simulink model "Simulink_TEP"  (R2024a)
settings: Solver=FixedStepAuto  StartTime=0.0  StopTime=5  FixedStep=1/3600  RelTol=1e-3
model workspace (MAT data in the model file):
  AD : Simulink.Parameter (value not decoded)
  AG : Simulink.Parameter (value not decoded)
  AH : Simulink.Parameter (value not decoded)
  AV : Simulink.Parameter (value not decoded)
  AVP : Simulink.Parameter (value not decoded)
  BCHL : Simulink.Parameter (value not decoded)
  BCHV : Simulink.Parameter (value not decoded)
  BD : Simulink.Parameter (value not decoded)
  BG : Simulink.Parameter (value not decoded)
  BH : Simulink.Parameter (value not decoded)
  BVP : Simulink.Parameter (value not decoded)
  CD : Simulink.Parameter (value not decoded)
  CG : Simulink.Parameter (value not decoded)
  CH : Simulink.Parameter (value not decoded)
  CVP : Simulink.Parameter (value not decoded)
  XMW : Simulink.Parameter (value not decoded)
symbols that are objects in the model workspace (value not decoded): AD, AG, AH, AV, AVP, BD, BG, BH, BVP, CD, CG, CH, CVP, XMW
undefined symbols (not defined in the file or in its folder): magnitude, SETPT, XMEAS, XMV
libraries: mylib x165, dspindex x17
(part 4 of 10)

== system Simulink_TEP/Subsystem/Braatz ==
  XMEAS : Inport
  " " : Subsystem  mask{Parameter1=XMV(1), Parameter2=XMEAS(2), SETPT1=3664.0, GAIN1=1.0, SI1=3, HIGH1=5811, Parameter1_copy=SETPT(1), Parameter2_copy=XMEAS(26), SETPT14=6.8820, GAIN14=8.3, TAUI14=3168.0/3600, SI14=360, HIGH14=100}
      mask prompts: Parameter1 "Manipulated Variable"; Parameter2 "Process Variable"; SETPT1 "Setpoint"; GAIN1 "Controller Gain"; SI1 "Sampling Interval"; HIGH1 "High Limit"; Parameter1_copy "Manipulated Variable"; Parameter2_copy "Process Variable"; SETPT14 "Setpoint"; GAIN14 "Controller Gain"; TAUI14 "Integral Time Constant"; SI14 "Sampling Interval"; HIGH14 "High Limit"
      mask DialogControl DescGroupVar Prompt: Control Variables
      mask DialogControl DescTextVar Prompt: Enter the control variables needed
      mask DialogControl ParameterGroupVar Prompt: Control 1
      mask DialogControl Container3 Prompt: Control 14
  " 1" : Subsystem  mask{Parameter1=XMV(2), Parameter2=XMEAS(3), SETPT2=4509.3, GAIN2=1.0, SI2=3, HIGH2=8354, Parameter1_copy=SETPT(2), Parameter2_copy=XMEAS(27), SETPT15=18.776, GAIN15=2.37, TAUI15=5069/3600, SI15=360, HIGH15=100}
      mask prompts: Parameter1 "Manipulated Variable"; Parameter2 "Process Variable"; SETPT2 "Setpoint"; GAIN2 "Controller Gain"; SI2 "Sampling Interval"; HIGH2 "High Limit"; Parameter1_copy "Manipulated Variable"; Parameter2_copy "Process Variable"; SETPT15 "Setpoint"; GAIN15 "Controller Gain"; TAUI15 "Integral Time Constant"; SI15 "Sampling Interval"; HIGH15 "High Limit"
      mask DialogControl DescGroupVar Prompt: Control Variables
      mask DialogControl DescTextVar Prompt: Enter the control variables needed
      mask DialogControl ParameterGroupVar Prompt: Control 2
      mask DialogControl Container3 Prompt: Control 15
  " 10" : Subsystem  mask{Parameter1=XMV(6), Parameter2=XMEAS(10), SETPT6=0.33712, GAIN6=1.22, SI6=3, HIGH6=1, Parameter1_copy=SETPT(6), Parameter2_copy=XMEAS(30), SETPT19=13.823, GAIN19=-83.2/5/3, TAUI19=6336/3600, SI19=360, HIGH19=26}
      mask prompts: Parameter1 "Manipulated Variable"; Parameter2 "Process Variable"; SETPT6 "Setpoint"; GAIN6 "Controller Gain"; SI6 "Sampling Interval"; HIGH6 "High Limit"; Parameter1_copy "Manipulated Variable"; Parameter2_copy "Process Variable"; SETPT19 "Setpoint"; GAIN19 "Controller Gain"; TAUI19 "Integral Time Constant"; SI19 "Sampling Interval"; HIGH19 "High Limit"
      mask DialogControl DescGroupVar Prompt: Control Variables
      mask DialogControl DescTextVar Prompt: Enter the control variables needed
      mask DialogControl ParameterGroupVar Prompt: Control 6
      mask DialogControl Container3 Prompt: Control 19
  " 2" : Subsystem  mask{Parameter1=XMV(3), Parameter2=XMEAS(1), SETPT3=0.25052, GAIN3=1.0, SI3=3, HIGH3=1.017, Parameter1_copy=SETPT(3), Parameter2_copy=XMEAS(23), SETPT13=32.188, GAIN13=18, TAUI13=3168.0/3600, SI13=360, HIGH13=100}
      mask prompts: Parameter1 "Manipulated Variable"; Parameter2 "Process Variable"; SETPT3 "Setpoint"; GAIN3 "Controller Gain"; SI3 "Sampling Interval"; HIGH3 "High Limit"; Parameter1_copy "Manipulated Variable"; Parameter2_copy "Process Variable"; SETPT13 "Setpoint"; GAIN13 "Controller Gain"; TAUI13 "Integral Time Constant"; SI13 "Sampling Interval"; HIGH13 "High Limit"
      mask DialogControl DescGroupVar Prompt: Control Variables
      mask DialogControl DescTextVar Prompt: Enter the control variables needed
      mask DialogControl ParameterGroupVar Prompt: Control 3
      mask DialogControl Container3 Prompt: Control 13
  " 3" : Subsystem  mask{Parameter1=XMV(4), Parameter2=XMEAS(4), SETPT4=9.3477, GAIN4=1.0, SI4=3, HIGH4=15.25, Parameter1_copy=SETPT(4), Parameter2_copy=XMEAS(8), SETPT17=75, GAIN17=11.1/10, TAUI17=3168.0/3600, SI17=3, HIGH17=50}
      mask prompts: Parameter1 "Manipulated Variable"; Parameter2 "Process Variable"; SETPT4 "Setpoint"; GAIN4 "Controller Gain"; SI4 "Sampling Interval"; HIGH4 "High Limit"; Parameter1_copy "Manipulated Variable"; Parameter2_copy "Process Variable"; SETPT17 "Setpoint"; GAIN17 "Controller Gain"; TAUI17 "Integral Time Constant"; SI17 "Sampling Interval"; HIGH17 "High Limit"
      mask DialogControl DescGroupVar Prompt: Control Variables
      mask DialogControl DescTextVar Prompt: Enter the control variables needed
      mask DialogControl ParameterGroupVar Prompt: Control 4
      mask DialogControl Container3 Prompt: Control 17
  " 4" : Subsystem  mask{Parameter1_copy=XMV(5), Parameter2_copy=XMEAS(5), SETPT5=26.902, GAIN5=-0.083, TAUI5=1/3600, SI5=3, HIGH5=53}
      mask prompts: Parameter1_copy "Manipulated Variable"; Parameter2_copy "Process Variable"; SETPT5 "Setpoint"; GAIN5 "Controller Gain"; TAUI5 "Integral Time Constant"; SI5 "Sampling Interval"; HIGH5 "High Limit"
      mask DialogControl DescGroupVar Prompt: Control Variables
      mask DialogControl DescTextVar Prompt: Enter the control variables needed
      mask DialogControl Container3 Prompt: Control 5
  " 5" : Subsystem  mask{Parameter1_copy=XMV(7), Parameter2_copy=XMEAS(12), SETPT7=50, GAIN7=-2.06, SI7=3, HIGH7=70}
      mask prompts: Parameter1_copy "Manipulated Variable"; Parameter2_copy "Process Variable"; SETPT7 "Setpoint"; GAIN7 "Controller Gain"; SI7 "Sampling Interval"; HIGH7 "High Limit"
      mask DialogControl DescGroupVar Prompt: Control Variables
      mask DialogControl DescTextVar Prompt: Enter the control variables needed
      mask DialogControl Container3 Prompt: Control 7
  " 6" : Subsystem  mask{Parameter1_copy=XMV(8), Parameter2_copy=XMEAS(15), SETPT8=50, GAIN8=-1.62, SI8=3, HIGH8=70}
      mask prompts: Parameter1_copy "Manipulated Variable"; Parameter2_copy "Process Variable"; SETPT8 "Setpoint"; GAIN8 "Controller Gain"; SI8 "Sampling Interval"; HIGH8 "High Limit"
      mask DialogControl DescGroupVar Prompt: Control Variables
      mask DialogControl DescTextVar Prompt: Enter the control variables needed
      mask DialogControl Container3 Prompt: Control 8
  " 7" : Subsystem  mask{Parameter1_copy=XMV(11), Parameter2_copy=XMEAS(17), SETPT11=22.949, GAIN11=1.09, TAUI11=2600/3600, SI11=3, HIGH11=46}
      mask prompts: Parameter1_copy "Manipulated Variable"; Parameter2_copy "Process Variable"; SETPT11 "Setpoint"; GAIN11 "Controller Gain"; TAUI11 "Integral Time Constant"; SI11 "Sampling Interval"; HIGH11 "High Limit"
      mask DialogControl DescGroupVar Prompt: Control Variables
      mask DialogControl DescTextVar Prompt: Enter the control variables needed
      mask DialogControl Container3 Prompt: Control 11
  " 8" : Subsystem  mask{Parameter1=XMV(10), Parameter2=XMEAS(21), SETPT10=94.599, GAIN10=-0.156*10, TAUI10=1452/3600, SI10=3, HIGH10=150, Parameter1_copy=SETPT(10), Parameter2_copy=XMEAS(9), SETPT18=120.4, GAIN18=2.83*10, TAUI18=982/3600, SI18=3, HIGH18=150}
      mask prompts: Parameter1 "Manipulated Variable"; Parameter2 "Process Variable"; SETPT10 "Setpoint"; GAIN10 "Controller Gain"; TAUI10 "Integral Time Constant"; SI10 "Sampling Interval"; HIGH10 "High Limit"; Parameter1_copy "Manipulated Variable"; Parameter2_copy "Process Variable"; SETPT18 "Setpoint"; GAIN18 "Controller Gain"; TAUI18 "Integral Time Constant"; SI18 "Sampling Interval"; HIGH18 "High Limit"
      mask DialogControl DescGroupVar Prompt: Control Variables
      mask DialogControl DescTextVar Prompt: Enter the control variables needed
      mask DialogControl ParameterGroupVar Prompt: Control 10
      mask DialogControl Container3 Prompt: Control 18
  " 9" : Subsystem  mask{Parameter1=XMV(9), Parameter2=XMEAS(19), SETPT9=230.31, GAIN9=0.41, SI9=3, HIGH9=460, Parameter1_copy=SETPT(9), Parameter2_copy=XMEAS(18), SETPT16=65.731, GAIN16=1.69/10, TAUI16=236/3600, SI16=3, HIGH16=130, Parameter1_copy_copy=SETPT(16), Parameter2_copy_copy=XMEAS(38), SETPT20=0.83570, GAIN20=-16.3/5, TAUI20=12408/3600, SI20=900, HIGH20=1.6}
      mask prompts: Parameter1 "Manipulated Variable"; Parameter2 "Process Variable"; SETPT9 "Setpoint"; GAIN9 "Controller Gain"; SI9 "Sampling Interval"; HIGH9 "High Limit"; Parameter1_copy "Manipulated Variable"; Parameter2_copy "Process Variable"; SETPT16 "Setpoint"; GAIN16 "Controller Gain"; TAUI16 "Integral Time Constant"; SI16 "Sampling Interval"; HIGH16 "High Limit"; Parameter1_copy_copy "Manipulated Variable"; Parameter2_copy_copy "Process Variable"; SETPT20 "Setpoint"; GAIN20 "Controller Gain"; TAUI20 "Integral Time Constant"; SI20 "Sampling Interval"; HIGH20 "High Limit"
      mask DialogControl DescGroupVar Prompt: Control Variables
      mask DialogControl DescTextVar Prompt: Enter the control variables needed
      mask DialogControl ParameterGroupVar Prompt: Control 9
      mask DialogControl Container3 Prompt: Control 16
      mask DialogControl Container3_copy Prompt: Control 20
  Bus Creator : BusCreator  Inputs=12
  Constant11 : Constant  Value=XMV12_0
  XMV : Outport  VectorParamsAs1DForOutWhenUnconnected=off
  wires:
  " "/1(XMV(1)) -> Bus Creator/1  "XMV(1)"
  " 1"/1(XMV(2)) -> Bus Creator/2  "XMV(2)"
  " 2"/1(XMV(3)) -> Bus Creator/3  "XMV(3)"
  " 3"/1(XMV(4)) -> Bus Creator/4  "XMV(4)"
  " 4"/1(XMV(5)) -> Bus Creator/5  "XMV(5)"
  " 10"/1(XMV(6)) -> Bus Creator/6  "XMV(6)"
  " 5"/1(XMV(7)) -> Bus Creator/7  "XMV(7)"
  " 6"/1(XMV(8)) -> Bus Creator/8  "XMV(8)"
  " 9"/1(XMV(9)) -> Bus Creator/9  "XMV(9)"
  " 8"/1(XMV(10)) -> Bus Creator/10  "XMV(10)"
  " 7"/1(XMV(11)) -> Bus Creator/11  "XMV(11)"
  Constant11/1 -> Bus Creator/12  "XMV(12)"
  Bus Creator/1 -> XMV/1
  XMEAS/1 -> " 5"/1(XMEAS), " 9"/1(XMEAS), " 8"/1(XMEAS), " 7"/1(XMEAS), " 6"/1(XMEAS), " 10"/1(XMEAS), " 4"/1(XMEAS), " 3"/1(XMEAS), " 2"/1(XMEAS), " 1"/1(XMEAS), " "/1(XMEAS)

== system Simulink_TEP/Subsystem/If Action Subsystem ==
  In1 : Inport
  Action Port : ActionPort  ActionPortLabel=if(u1 == 1)
  Out1 : Outport  VectorParamsAs1DForOutWhenUnconnected=off
  wires:
  In1/1 -> Out1/1

== system Simulink_TEP/Subsystem/If Action Subsystem1 ==
  In1 : Inport
  Action Port : ActionPort  ActionPortLabel=elseif(u2 == 1)
  Out1 : Outport  VectorParamsAs1DForOutWhenUnconnected=off
  wires:
  In1/1 -> Out1/1

== system Simulink_TEP/Subsystem/If Action Subsystem2 ==
  In1 : Inport
  Action Port : ActionPort  ActionPortLabel=elseif( u3 == 1)
  Out1 : Outport  VectorParamsAs1DForOutWhenUnconnected=off
  wires:
  In1/1 -> Out1/1

== system Simulink_TEP/Subsystem/Open loop ==
  Bus Creator : BusCreator  Inputs=12
  Constant : Constant  Value=XMV1_0
  Constant1 : Constant  Value=XMV2_0
  Constant10 : Constant  Value=XMV11_0
  Constant11 : Constant  Value=XMV12_0
  Constant2 : Constant  Value=XMV3_0
  Constant3 : Constant  Value=XMV4_0
  Constant4 : Constant  Value=XMV5_0
  Constant5 : Constant  Value=XMV6_0
  Constant6 : Constant  Value=XMV7_0
  Constant7 : Constant  Value=XMV8_0
  Constant8 : Constant  Value=XMV9_0
  Constant9 : Constant  Value=XMV10_0
  XMV : Outport  VectorParamsAs1DForOutWhenUnconnected=off
  wires:
  Constant5/1 -> Bus Creator/6  "XMV(6)"
  Constant1/1 -> Bus Creator/2  "XMV(2)"
  Constant4/1 -> Bus Creator/5  "XMV(5)"
  Constant3/1 -> Bus Creator/4  "XMV(4)"
  Constant2/1 -> Bus Creator/3  "XMV(3)"
  Constant11/1 -> Bus Creator/12  "XMV(12)"
  Constant10/1 -> Bus Creator/11  "XMV(11)"
  Constant/1 -> Bus Creator/1  "XMV(1)"
  Constant9/1 -> Bus Creator/10  "XMV(10)"
  Constant8/1 -> Bus Creator/9  "XMV(9)"
  Constant6/1 -> Bus Creator/7  "XMV(7)"
  Bus Creator/1 -> XMV/1
  Constant7/1 -> Bus Creator/8  "XMV(8)"

== system Simulink_TEP/Subsystem/Ricker ==
  Bus Creator : BusCreator  Inputs=12
  Constant : Constant  Value=XMV1_0
  Constant1 : Constant  Value=XMV2_0
  Constant10 : Constant  Value=XMV11_0
  Constant11 : Constant  Value=XMV12_0
  Constant2 : Constant  Value=XMV3_0
  Constant3 : Constant  Value=XMV4_0
  Constant4 : Constant  Value=XMV5_0
  Constant5 : Constant  Value=XMV6_0
  Constant6 : Constant  Value=XMV7_0
  Constant7 : Constant  Value=XMV8_0
  Constant8 : Constant  Value=XMV9_0
  Constant9 : Constant  Value=XMV10_0
  XMV : Outport  VectorParamsAs1DForOutWhenUnconnected=off
  wires:
  Constant5/1 -> Bus Creator/6  "XMV(6)"
  Constant1/1 -> Bus Creator/2  "XMV(2)"
  Constant4/1 -> Bus Creator/5  "XMV(5)"
  Constant3/1 -> Bus Creator/4  "XMV(4)"
  Constant2/1 -> Bus Creator/3  "XMV(3)"
  Constant11/1 -> Bus Creator/12  "XMV(12)"
  Constant10/1 -> Bus Creator/11  "XMV(11)"
  Constant/1 -> Bus Creator/1  "XMV(1)"
  Constant9/1 -> Bus Creator/10  "XMV(10)"
  Constant8/1 -> Bus Creator/9  "XMV(9)"
  Constant6/1 -> Bus Creator/7  "XMV(7)"
  Bus Creator/1 -> XMV/1
  Constant7/1 -> Bus Creator/8  "XMV(8)"

== system Simulink_TEP/Subsystem/Subsystem ==
  OPL : Inport
  B : Inport  Port=2
  R : Inport  Port=3
  Assertion : Assertion  AssertionFailFcn=|  StopWhenAssertionFail=off
      | set_param(bdroot,'SimulationCommand','stop'),
      | disp(sprintf('\nSimulation stoped.')), msgbox({'Simulation will not run';'More than one loop selected'}, 'Shutdown','error')
  Constant3 : Constant  Value=2
  Relational Operator : RelationalOperator  Operator=<  OutDataTypeStr=boolean  RndMeth=Simplest  InputSameDT=off
  Sum of Elements : Sum  Inputs=+++
  wires:
  Sum of Elements/1 -> Relational Operator/1
  R/1 -> Sum of Elements/3
  OPL/1 -> Sum of Elements/1
  Relational Operator/1 -> Assertion/1
  Constant3/1 -> Relational Operator/2
  B/1 -> Sum of Elements/2

== system Simulink_TEP/Subsystem1/Subsystem ==
  Stream 6 : Inport
  Bus Creator : BusCreator  Inputs=2
  Bus Selector : BusSelector  OutputSignals=signal1.Phase,signal1.TST(6) = TST(7),signal1.XST(I;6) = XST(I;7),PTV,signal1.FTM(6) = FTM(7)
  Exergy Molar Flow : mylib/Exergy Molar Flow  SystemSampleTime=-1  VariantActivationTime=update diagram  AllowFlexibleInterface=on  Latency=0  AutoFrameSizeCalculation=off
  B1 : Outport  VectorParamsAs1DForOutWhenUnconnected=off
  wires:
  Bus Selector/4 -> Exergy Molar Flow/4  "<PTV>"
  Exergy Molar Flow/2 -> Bus Creator/2  "Bph1"
  Bus Selector/5 -> Exergy Molar Flow/5  "<FTM(6) = FTM(7)>"
  Bus Selector/2 -> Exergy Molar Flow/2  "<TST(6) = TST(7)>"
  Stream 6/1 -> Bus Selector/1
  Bus Creator/1 -> B1/1  "B1"
  Bus Selector/3 -> Exergy Molar Flow/3  "<XST(I;6) = XST(I;7)>"
  Exergy Molar Flow/1 -> Bus Creator/1  "Bch1"
  Bus Selector/1 -> Exergy Molar Flow/1  "<Phase>"

== system Simulink_TEP/Subsystem1/Subsystem1 ==
  Stream 8 : Inport
  Bus Creator1 : BusCreator  Inputs=2
  Bus Selector : BusSelector  OutputSignals=signal1.Phase,signal1.TST(8),signal1.XST(I;8),PTR,signal1.FTM(8)
  Exergy Molar Flow : mylib/Exergy Molar Flow  SystemSampleTime=-1  VariantActivationTime=update diagram  AllowFlexibleInterface=on  Latency=0  AutoFrameSizeCalculation=off
  B2 : Outport  VectorParamsAs1DForOutWhenUnconnected=off
  wires:
  Bus Selector/4 -> Exergy Molar Flow/4  "<PTR>"
  Bus Selector/5 -> Exergy Molar Flow/5  "<FTM(8)>"
  Bus Selector/2 -> Exergy Molar Flow/2  "<TST(8)>"
  Stream 8/1 -> Bus Selector/1
  Bus Selector/3 -> Exergy Molar Flow/3  "<XST(I;8)>"
  Bus Selector/1 -> Exergy Molar Flow/1  "<Phase>"
  Exergy Molar Flow/2 -> Bus Creator1/2  "Bph2"
  Bus Creator1/1 -> B2/1  "B2"
  Exergy Molar Flow/1 -> Bus Creator1/1  "Bch2"

== system Simulink_TEP/Subsystem1/Subsystem2 ==
  Stream 9 : Inport
  Bus Creator2 : BusCreator  Inputs=2
  Bus Selector : BusSelector  OutputSignals=signal2.Phase,signal2.TST(9),signal2.XST(I;9),PTS,signal2.FTM(9)
  Exergy Molar Flow : mylib/Exergy Molar Flow  SystemSampleTime=-1  VariantActivationTime=update diagram  AllowFlexibleInterface=on  Latency=0  AutoFrameSizeCalculation=off
  B3 : Outport  VectorParamsAs1DForOutWhenUnconnected=off
  wires:
  Bus Selector/4 -> Exergy Molar Flow/4  "<PTS>"
  Bus Selector/5 -> Exergy Molar Flow/5  "<FTM(9)>"
  Bus Selector/2 -> Exergy Molar Flow/2  "<TST(9)>"
  Stream 9/1 -> Bus Selector/1
  Bus Selector/3 -> Exergy Molar Flow/3  "<XST(I;9)>"
  Bus Selector/1 -> Exergy Molar Flow/1  "<Phase>"
  Exergy Molar Flow/1 -> Bus Creator2/1  "Bch3"
  Exergy Molar Flow/2 -> Bus Creator2/2  "Bph3"
  Bus Creator2/1 -> B3/1  "B3"

== system Simulink_TEP/Subsystem1/Subsystem3 ==
  Stream 10 : Inport
  Bus Creator3 : BusCreator  Inputs=2
  Bus Selector : BusSelector  OutputSignals=signal1.Phase,signal1.TST(10),signal1.XST(I;10),PTS,signal1.FTM(10)
  Exergy Molar Flow : mylib/Exergy Molar Flow  SystemSampleTime=-1  VariantActivationTime=update diagram  AllowFlexibleInterface=on  Latency=0  AutoFrameSizeCalculation=off
  B4 : Outport  VectorParamsAs1DForOutWhenUnconnected=off
  wires:
  Bus Selector/4 -> Exergy Molar Flow/4  "<PTS>"
  Bus Selector/5 -> Exergy Molar Flow/5  "<FTM(10)>"
  Bus Selector/2 -> Exergy Molar Flow/2  "<TST(10)>"
  Stream 10/1 -> Bus Selector/1
  Bus Selector/3 -> Exergy Molar Flow/3  "<XST(I;10)>"
  Bus Selector/1 -> Exergy Molar Flow/1  "<Phase>"
  Exergy Molar Flow/2 -> Bus Creator3/2  "Bph4"
  Exergy Molar Flow/1 -> Bus Creator3/1  "Bch4"
  Bus Creator3/1 -> B4/1  "B4"

== system Simulink_TEP/Subsystem1/Subsystem4 ==
  Stream 11 : Inport
  Bus Creator4 : BusCreator  Inputs=2
  Bus Selector : BusSelector  OutputSignals=signal1.Phase,signal1.TST(11),signal1.XST(I;11),PTS,signal1.FTM(11)
  Exergy Molar Flow : mylib/Exergy Molar Flow  SystemSampleTime=-1  VariantActivationTime=update diagram  AllowFlexibleInterface=on  Latency=0  AutoFrameSizeCalculation=off
  B5 : Outport  VectorParamsAs1DForOutWhenUnconnected=off
  wires:
  Bus Selector/4 -> Exergy Molar Flow/4  "<PTS>"
  Bus Selector/5 -> Exergy Molar Flow/5  "<FTM(11)>"
  Bus Selector/2 -> Exergy Molar Flow/2  "<TST(11)>"
  Stream 11/1 -> Bus Selector/1
  Bus Selector/3 -> Exergy Molar Flow/3  "<XST(I;11)>"
  Bus Selector/1 -> Exergy Molar Flow/1  "<Phase>"
  Exergy Molar Flow/1 -> Bus Creator4/1  "Bch5"
  Bus Creator4/1 -> B5/1  "B5"
  Exergy Molar Flow/2 -> Bus Creator4/2  "Bph5"

== system Simulink_TEP/Subsystem1/Subsystem5 ==
  Stream 5 : Inport
  Bus Creator5 : BusCreator  Inputs=2
  Bus Selector : BusSelector  OutputSignals=Phase,TST(5),XST(I;5),PTV,FTM(5)
  Exergy Molar Flow : mylib/Exergy Molar Flow  SystemSampleTime=-1  VariantActivationTime=update diagram  AllowFlexibleInterface=on  Latency=0  AutoFrameSizeCalculation=off
  B6 : Outport  VectorParamsAs1DForOutWhenUnconnected=off
  wires:
  Bus Selector/4 -> Exergy Molar Flow/4  "<PTV>"
  Bus Selector/5 -> Exergy Molar Flow/5  "<FTM(5)>"
  Bus Selector/2 -> Exergy Molar Flow/2  "<TST(5)>"
  Stream 5/1 -> Bus Selector/1
  Bus Selector/3 -> Exergy Molar Flow/3  "<XST(I;5)>"
  Bus Selector/1 -> Exergy Molar Flow/1  "<Phase>"
  Bus Creator5/1 -> B6/1  "B6"
  Exergy Molar Flow/1 -> Bus Creator5/1  "Bch6"
  Exergy Molar Flow/2 -> Bus Creator5/2  "Bph6"

== system Simulink_TEP/Subsystem1/Subsystem6 ==
  Stream 13 : Inport
  Bus Creator6 : BusCreator  Inputs=2
  Bus Selector : BusSelector  OutputSignals=Phase,TST(13),XST(I;13),PTC,FTM(13)
  Exergy Molar Flow : mylib/Exergy Molar Flow  SystemSampleTime=-1  VariantActivationTime=update diagram  AllowFlexibleInterface=on  Latency=0  AutoFrameSizeCalculation=off
  B7 : Outport  VectorParamsAs1DForOutWhenUnconnected=off
  wires:
  Bus Selector/4 -> Exergy Molar Flow/4  "<PTC>"
  Bus Selector/5 -> Exergy Molar Flow/5  "<FTM(13)>"
  Bus Selector/2 -> Exergy Molar Flow/2  "<TST(13)>"
  Stream 13/1 -> Bus Selector/1
  Bus Selector/3 -> Exergy Molar Flow/3  "<XST(I;13)>"
  Bus Selector/1 -> Exergy Molar Flow/1  "<Phase>"
  Bus Creator6/1 -> B7/1  "B7"
  Exergy Molar Flow/2 -> Bus Creator6/2  "Bph7"
  Exergy Molar Flow/1 -> Bus Creator6/1  "Bch7"

== system Simulink_TEP/Valve/FTM(1) Total molar flow of Stream 1 lb-mol//h ==
  VPOS(1) : Inport
  VRNG(1) : Inport  Port=2
  " " : Product  Inputs=**/
  Constant : Constant  Value=100
  FTM(1) : Outport  PortDimensions=1  VectorParamsAs1DForOutWhenUnconnected=off
  wires:
  VRNG(1)/1 -> " "/2
  Constant/1 -> " "/3
  VPOS(1)/1 -> " "/1
  " "/1 -> FTM(1)/1

== system Simulink_TEP/Valve/Position of Valve 1 % ==
  Bus Selector : BusSelector  OutputSignals=XMV(1)
  Control valve : mylib/Control valve  SystemSampleTime=-1  VariantActivationTime=update diagram  AllowFlexibleInterface=on  Latency=0  AutoFrameSizeCalculation=off
  Divide : Product  Inputs=*/
  IVST(1) : Constant  Value=0
  Subtract : Sum  Inputs=+-
  VTAU(1) : Constant  Value=8/3600
  YP(39) : Integrator  InitialConditionSource=external
  YY(39) : Constant  Value=63.05263039
  "YY(39) " : Outport  VectorParamsAs1DForOutWhenUnconnected=off
  wires:
  YP(39)/1 -> "YY(39) "/1, Subtract/2  "VPOS(1)"
  YY(39)/1 -> YP(39)/2
  Subtract/1 -> Divide/1
  VTAU(1)/1 -> Divide/2
  Divide/1 -> YP(39)/1
  Control valve/1 -> Subtract/1
  [XMV] -> Bus Selector/1
  Bus Selector/1 -> Control valve/1  "<XMV(1)>"
  IVST(1)/1 -> Control valve/2

== system Simulink_TEP/Valve 2/FTM(2) Total molar flow of Stream 2 lb-mol//h ==
  VPOS(2) : Inport
  VRNG(2) : Inport  Port=2
  " " : Product  Inputs=**/
  Constant : Constant  Value=100
  FTM(2) : Outport  PortDimensions=1  VectorParamsAs1DForOutWhenUnconnected=off
  wires:
  VRNG(2)/1 -> " "/2
  Constant/1 -> " "/3
  VPOS(2)/1 -> " "/1
  " "/1 -> FTM(2)/1

== system Simulink_TEP/Valve 2/Position of Valve 2 % ==
  Bus Selector : BusSelector  OutputSignals=XMV(2)
  Control valve : mylib/Control valve  SystemSampleTime=-1  VariantActivationTime=update diagram  AllowFlexibleInterface=on  Latency=0  AutoFrameSizeCalculation=off
  Divide : Product  Inputs=*/
  IVST(2) : Constant  Value=0
  Subtract : Sum  Inputs=+-
  VTAU(2) : Constant  Value=8/3600
  YP(40) : Integrator  InitialConditionSource=external
  YY(40) : Constant  Value=53.97970677
  "YY(40)  " : Outport  VectorParamsAs1DForOutWhenUnconnected=off
  wires:
  Control valve/1 -> Subtract/1
  Subtract/1 -> Divide/1
  VTAU(2)/1 -> Divide/2
  Divide/1 -> YP(40)/1
  YP(40)/1 -> Subtract/2, "YY(40)  "/1  "VPOS(2)"
  YY(40)/1 -> YP(40)/2
  [XMV] -> Bus Selector/1
  Bus Selector/1 -> Control valve/1  "<XMV(2)>"
  IVST(2)/1 -> Control valve/2

== system Simulink_TEP/Valve 3/FTM(3) Total molar flow of Stream 3 lb-mol//h ==
  VPOS(3) : Inport
  VRNG(3) : Inport  Port=2
  " " : Product  Inputs=***/
  Bus Selector : BusSelector  OutputSignals=IDV(6)
  Constant : Constant  Value=100
  Constant1 : Constant
  Display : Display
  Display1 : Display
  Subtract : Sum  Inputs=+-
  FTM(3) : Outport  PortDimensions=1  VectorParamsAs1DForOutWhenUnconnected=off
  wires:
  VPOS(3)/1 -> " "/1
  " "/1 -> Display/1, FTM(3)/1
  Constant1/1 -> Subtract/1
  [IDV] -> Bus Selector/1
  Constant/1 -> " "/4
  Subtract/1 -> Display1/1, " "/2
  VRNG(3)/1 -> " "/3
  Bus Selector/1 -> Subtract/2  "<IDV(6)>"

== system Simulink_TEP/Valve 3/Position of Valve 3 % ==
  Bus Selector : BusSelector  OutputSignals=XMV(3)
  Control valve : mylib/Control valve  SystemSampleTime=-1  VariantActivationTime=update diagram  AllowFlexibleInterface=on  Latency=0  AutoFrameSizeCalculation=off
  Divide : Product  Inputs=*/
  IVST(3) : Constant  Value=0
  Subtract : Sum  Inputs=+-
  VTAU(3) : Constant  Value=6/3600
  YP(41) : Integrator  InitialConditionSource=external
  YY(41) : Constant  Value=24.64355755
  "YY(41) " : Outport  VectorParamsAs1DForOutWhenUnconnected=off
  wires:
  Control valve/1 -> Subtract/1
  Subtract/1 -> Divide/1
  VTAU(3)/1 -> Divide/2
  Divide/1 -> YP(41)/1
  YP(41)/1 -> Subtract/2, "YY(41) "/1  "VPOS(3)"
  YY(41)/1 -> YP(41)/2
  [XMV] -> Bus Selector/1
  Bus Selector/1 -> Control valve/1  "<XMV(3)>"
  IVST(3)/1 -> Control valve/2

== system Simulink_TEP/Valve 4/FTM(4) Total molar flow of Stream 4 lb-mol//h ==
  VPOS(4) : Inport
  VRNG(4) : Inport  Port=2
  " " : Product  Inputs=***/
  Add : Sum
  Bus Selector : BusSelector  OutputSignals=IDV(7)
  Constant : Constant
  Constant1 : Constant  Value=0.2
  Constant3 : Constant  Value=100
  Constant4 : Constant  Value=1e-10
  Product1 : Product
  Subtract : Sum  Inputs=+-
  FTM(4) : Outport  PortDimensions=1  VectorParamsAs1DForOutWhenUnconnected=off
  wires:
  Add/1 -> FTM(4)/1
  Constant4/1 -> Add/2
  " "/1 -> Add/1
  VPOS(4)/1 -> " "/1
  Bus Selector/1 -> Product1/1  "<IDV(7)>"
  Product1/1 -> Subtract/2
  Constant1/1 -> Product1/2
  Constant/1 -> Subtract/1
  Constant3/1 -> " "/4
  VRNG(4)/1 -> " "/3
  Subtract/1 -> " "/2
  [IDV] -> Bus Selector/1

== system Simulink_TEP/Valve 4/Position of Valve 4 % ==
  Bus Selector : BusSelector  OutputSignals=XMV(4)
  Control valve : mylib/Control valve  SystemSampleTime=-1  VariantActivationTime=update diagram  AllowFlexibleInterface=on  Latency=0  AutoFrameSizeCalculation=off
  Divide : Product  Inputs=*/
  IVST(4) : Constant  Value=0
  Subtract : Sum  Inputs=+-
  VTAU(4) : Constant  Value=9/3600
  YP(42) : Integrator  InitialConditionSource=external
  YY(42) : Constant  Value=61.30192144
  "YY(42) " : Outport  VectorParamsAs1DForOutWhenUnconnected=off
  wires:
  Control valve/1 -> Subtract/1
  Subtract/1 -> Divide/1
  VTAU(4)/1 -> Divide/2
  Divide/1 -> YP(42)/1
  YP(42)/1 -> Subtract/2, "YY(42) "/1  "VPOS(4)"
  YY(42)/1 -> YP(42)/2
  [XMV] -> Bus Selector/1
  Bus Selector/1 -> Control valve/1  "<XMV(4)>"
  IVST(4)/1 -> Control valve/2

== system Simulink_TEP/Compressor/Subsystem/If Action Subsystem ==
  In1 : Inport
  Action Port : ActionPort  ActionPortLabel=if(u1 < 1)
  Out1 : Outport  VectorParamsAs1DForOutWhenUnconnected=off
  wires:
  In1/1 -> Out1/1

== system Simulink_TEP/Compressor/Subsystem/If Action Subsystem1 ==
  In1 : Inport
  Action Port : ActionPort  ActionPortLabel=elseif(u1>1.3)
  Out1 : Outport  VectorParamsAs1DForOutWhenUnconnected=off
  wires:
  In1/1 -> Out1/1

== system Simulink_TEP/Compressor/Subsystem/If Action Subsystem2 ==
  In1 : Inport
  Action Port : ActionPort  ActionPortLabel=else
  Out1 : Outport  VectorParamsAs1DForOutWhenUnconnected=off
  wires:
  In1/1 -> Out1/1

== system Simulink_TEP/Condenser/Subsystem1/TCWS ==
  Add : Sum
  Bus Selector : BusSelector  OutputSignals=TESUB8(6)
  Bus Selector1 : BusSelector  OutputSignals=IDV(5)
  Constant : Constant  Value=5
  Product1 : Product
  TCWS : Outport  VectorParamsAs1DForOutWhenUnconnected=off
  wires:
  Constant/1 -> Product1/2
  Bus Selector/1 -> Add/1  "<TESUB8(6)>"
  Bus Selector1/1 -> Product1/1  "<IDV(5)>"
  [TESUB8] -> Bus Selector/1
  Product1/1 -> Add/2
  [IDV] -> Bus Selector1/1
  Add/1 -> TCWS/1

== system Simulink_TEP/Disturbances/Subsystem1/Subsystem2 ==
  IDVWLK : Inport
  DIST : Inport  Port=2
  Bus Selector : BusSelector  OutputSignals=TNEXT
  Bus Selector1 : BusSelector  OutputSignals=TESUB7_2
  Clock : Clock
  If : If  NumInputs=2  IfExpression=u1 == 0  ElseIfExpressions=u1 >= u2  ShowElse=off
  If Action Subsystem : Subsystem  TreatAsAtomicUnit=on
  If Action Subsystem1 : Subsystem  TreatAsAtomicUnit=on
  Merge : Merge
  DIST_NEW : Outport  VectorParamsAs1DForOutWhenUnconnected=off
  wires:
  Clock/1 -> If/1
  If/1 -> If Action Subsystem1/Action
  If/2 -> If Action Subsystem/Action
  Bus Selector/1 -> If/2  "<TNEXT>"
  If Action Subsystem/1(DIST_NEW) -> Merge/2
  IDVWLK/1 -> If Action Subsystem/1(IDWLK)
  If Action Subsystem1/1(DIST) -> Merge/1
  DIST/1 -> Bus Selector/1, If Action Subsystem/2("DIST ")
  Merge/1 -> DIST_NEW/1
  Bus Selector1/1 -> If Action Subsystem/3(TESUB7)  "<TESUB7_2>"
  [TESUB7] -> Bus Selector1/1

== system Simulink_TEP/Disturbances/Subsystem10/Subsystem3 ==
  IDVWLK : Inport
  DIST : Inport  Port=2
  Bus Selector : BusSelector  OutputSignals=TNEXT
  Bus Selector1 : BusSelector  OutputSignals=TESUB7_10
  Clock : Clock
  If : If  NumInputs=2  IfExpression=u1 == 0  ElseIfExpressions=u1 >= u2  ShowElse=off
  If Action Subsystem : Subsystem  TreatAsAtomicUnit=on
  If Action Subsystem1 : Subsystem  TreatAsAtomicUnit=on
  Merge : Merge
  DIST_NEW : Outport  VectorParamsAs1DForOutWhenUnconnected=off
  SWLK : Outport  Port=2  VectorParamsAs1DForOutWhenUnconnected=off
  wires:
  Clock/1 -> If/1
  If/1 -> If Action Subsystem1/Action
  If/2 -> If Action Subsystem/Action
  Bus Selector/1 -> If/2  "<TNEXT>"
  If Action Subsystem/1(DIST_NEW) -> Merge/2
  IDVWLK/1 -> If Action Subsystem/1(IDWLK)
  If Action Subsystem1/1(DIST) -> Merge/1
  DIST/1 -> Bus Selector/1, If Action Subsystem/2("DIST ")
  Merge/1 -> DIST_NEW/1
  Bus Selector1/1 -> If Action Subsystem/3(TESUB7)  "<TESUB7_10>"
  [TESUB7_2] -> Bus Selector1/1
  If Action Subsystem/2(SWLK) -> SWLK/1

== system Simulink_TEP/Disturbances/Subsystem11/Subsystem3 ==
  IDVWLK : Inport
  DIST : Inport  Port=2
  Bus Selector : BusSelector  OutputSignals=TNEXT
  Bus Selector1 : BusSelector  OutputSignals=TESUB7_11
  Clock : Clock
  If : If  NumInputs=2  IfExpression=u1 == 0  ElseIfExpressions=u1 >= u2  ShowElse=off
  If Action Subsystem : Subsystem  TreatAsAtomicUnit=on
  If Action Subsystem1 : Subsystem  TreatAsAtomicUnit=on
  Merge : Merge
  DIST_NEW : Outport  VectorParamsAs1DForOutWhenUnconnected=off
  SWLK : Outport  Port=2  VectorParamsAs1DForOutWhenUnconnected=off
  wires:
  Clock/1 -> If/1
  If/1 -> If Action Subsystem1/Action
  If/2 -> If Action Subsystem/Action
  Bus Selector/1 -> If/2  "<TNEXT>"
  If Action Subsystem/1(DIST_NEW) -> Merge/2
  IDVWLK/1 -> If Action Subsystem/1(IDWLK)
  If Action Subsystem1/1(DIST) -> Merge/1
  DIST/1 -> Bus Selector/1, If Action Subsystem/2("DIST ")
  Merge/1 -> DIST_NEW/1
  Bus Selector1/1 -> If Action Subsystem/3(TESUB7)  "<TESUB7_11>"
  [TESUB7_2] -> Bus Selector1/1
  If Action Subsystem/2(SWLK) -> SWLK/1

== system Simulink_TEP/Disturbances/Subsystem12/Subsystem3 ==
  IDVWLK : Inport
  DIST : Inport  Port=2
  Bus Selector : BusSelector  OutputSignals=TNEXT
  Bus Selector1 : BusSelector  OutputSignals=TESUB7_12
  Clock : Clock
  If : If  NumInputs=2  IfExpression=u1 == 0  ElseIfExpressions=u1 >= u2  ShowElse=off
  If Action Subsystem : Subsystem  TreatAsAtomicUnit=on
  If Action Subsystem1 : Subsystem  TreatAsAtomicUnit=on
  Merge : Merge
  DIST_NEW : Outport  VectorParamsAs1DForOutWhenUnconnected=off
  SWLK : Outport  Port=2  VectorParamsAs1DForOutWhenUnconnected=off
  wires:
  Clock/1 -> If/1
  If/1 -> If Action Subsystem1/Action
  If/2 -> If Action Subsystem/Action
  Bus Selector/1 -> If/2  "<TNEXT>"
  If Action Subsystem/1(DIST_NEW) -> Merge/2
  IDVWLK/1 -> If Action Subsystem/1(IDWLK)
  If Action Subsystem1/1(DIST) -> Merge/1
  DIST/1 -> Bus Selector/1, If Action Subsystem/2("DIST ")
  Merge/1 -> DIST_NEW/1
  Bus Selector1/1 -> If Action Subsystem/3(TESUB7)  "<TESUB7_12>"
  [TESUB7_2] -> Bus Selector1/1
  If Action Subsystem/2(SWLK) -> SWLK/1

== system Simulink_TEP/Disturbances/Subsystem2/Subsystem ==
  IDVWLK : Inport
  DIST : Inport  Port=2
  Bus Selector : BusSelector  OutputSignals=TNEXT
  Bus Selector1 : BusSelector  OutputSignals=TESUB7_1
  Clock : Clock
  If : If  NumInputs=2  IfExpression=u1 == 0  ElseIfExpressions=u1 >= u2  ShowElse=off
  If Action Subsystem : Subsystem  TreatAsAtomicUnit=on
  If Action Subsystem1 : Subsystem  TreatAsAtomicUnit=on
  Merge : Merge
  DIST_NEW : Outport  VectorParamsAs1DForOutWhenUnconnected=off
  wires:
  Clock/1 -> If/1
  If/1 -> If Action Subsystem1/Action
  If/2 -> If Action Subsystem/Action
  Bus Selector/1 -> If/2  "<TNEXT>"
  If Action Subsystem/1(DIST_NEW) -> Merge/2
  IDVWLK/1 -> If Action Subsystem/1(IDWLK)
  If Action Subsystem1/1(DIST) -> Merge/1
  DIST/1 -> Bus Selector/1, If Action Subsystem/2("DIST ")
  Merge/1 -> DIST_NEW/1
  Bus Selector1/1 -> If Action Subsystem/3(TESUB7)  "<TESUB7_1>"
  [TESUB7] -> Bus Selector1/1

== system Simulink_TEP/Disturbances/Subsystem3/Subsystem2 ==
  IDVWLK : Inport
  DIST : Inport  Port=2
  Bus Selector : BusSelector  OutputSignals=TNEXT
  Bus Selector1 : BusSelector  OutputSignals=TESUB7_3
  Clock : Clock
  If : If  NumInputs=2  IfExpression=u1 == 0  ElseIfExpressions=u1 >= u2  ShowElse=off
  If Action Subsystem : Subsystem  TreatAsAtomicUnit=on
  If Action Subsystem1 : Subsystem  TreatAsAtomicUnit=on
  Merge : Merge
  DIST_NEW : Outport  VectorParamsAs1DForOutWhenUnconnected=off
  wires:
  Clock/1 -> If/1
  If/1 -> If Action Subsystem1/Action
  If/2 -> If Action Subsystem/Action
  Bus Selector/1 -> If/2  "<TNEXT>"
  If Action Subsystem/1(DIST_NEW) -> Merge/2
  IDVWLK/1 -> If Action Subsystem/1(IDWLK)
  If Action Subsystem1/1(DIST) -> Merge/1
  DIST/1 -> Bus Selector/1, If Action Subsystem/2("DIST ")
  Merge/1 -> DIST_NEW/1
  Bus Selector1/1 -> If Action Subsystem/3(TESUB7)  "<TESUB7_3>"
  [TESUB7] -> Bus Selector1/1

== system Simulink_TEP/Disturbances/Subsystem4/Subsystem2 ==
  IDVWLK : Inport
  DIST : Inport  Port=2
  Bus Selector : BusSelector  OutputSignals=TNEXT
  Bus Selector1 : BusSelector  OutputSignals=TESUB7_4
  Clock : Clock
  If : If  NumInputs=2  IfExpression=u1 == 0  ElseIfExpressions=u1 >= u2  ShowElse=off
  If Action Subsystem : Subsystem  TreatAsAtomicUnit=on
  If Action Subsystem1 : Subsystem  TreatAsAtomicUnit=on
  Merge : Merge
  DIST_NEW : Outport  VectorParamsAs1DForOutWhenUnconnected=off
  wires:
  Clock/1 -> If/1
  If/1 -> If Action Subsystem1/Action
  If/2 -> If Action Subsystem/Action
  Bus Selector/1 -> If/2  "<TNEXT>"
  If Action Subsystem/1(DIST_NEW) -> Merge/2
  IDVWLK/1 -> If Action Subsystem/1(IDWLK)
  If Action Subsystem1/1(DIST) -> Merge/1
  DIST/1 -> Bus Selector/1, If Action Subsystem/2("DIST ")
  Merge/1 -> DIST_NEW/1
  Bus Selector1/1 -> If Action Subsystem/3(TESUB7)  "<TESUB7_4>"
  [TESUB7] -> Bus Selector1/1

== system Simulink_TEP/Disturbances/Subsystem5/Subsystem2 ==
  IDVWLK : Inport
  DIST : Inport  Port=2
  Bus Selector : BusSelector  OutputSignals=TNEXT
  Bus Selector1 : BusSelector  OutputSignals=TESUB7_5
  Clock : Clock
  If : If  NumInputs=2  IfExpression=u1 == 0  ElseIfExpressions=u1 >= u2  ShowElse=off
  If Action Subsystem : Subsystem  TreatAsAtomicUnit=on
  If Action Subsystem1 : Subsystem  TreatAsAtomicUnit=on
  Merge : Merge
  DIST_NEW : Outport  VectorParamsAs1DForOutWhenUnconnected=off
  wires:
  Clock/1 -> If/1
  If/1 -> If Action Subsystem1/Action
  If/2 -> If Action Subsystem/Action
  Bus Selector/1 -> If/2  "<TNEXT>"
  If Action Subsystem/1(DIST_NEW) -> Merge/2
  IDVWLK/1 -> If Action Subsystem/1(IDWLK)
  If Action Subsystem1/1(DIST) -> Merge/1
  DIST/1 -> Bus Selector/1, If Action Subsystem/2("DIST ")
  Merge/1 -> DIST_NEW/1
  Bus Selector1/1 -> If Action Subsystem/3(TESUB7)  "<TESUB7_5>"
  [TESUB7] -> Bus Selector1/1

== system Simulink_TEP/Disturbances/Subsystem6/Subsystem2 ==
  IDVWLK : Inport
  DIST : Inport  Port=2
  Bus Selector : BusSelector  OutputSignals=TNEXT
  Bus Selector1 : BusSelector  OutputSignals=TESUB7_6
  Clock : Clock
  If : If  NumInputs=2  IfExpression=u1 == 0  ElseIfExpressions=u1 >= u2  ShowElse=off
  If Action Subsystem : Subsystem  TreatAsAtomicUnit=on
  If Action Subsystem1 : Subsystem  TreatAsAtomicUnit=on
  Merge : Merge
  DIST_NEW : Outport  VectorParamsAs1DForOutWhenUnconnected=off
  wires:
  Clock/1 -> If/1
  If/1 -> If Action Subsystem1/Action
  If/2 -> If Action Subsystem/Action
  Bus Selector/1 -> If/2  "<TNEXT>"
  If Action Subsystem/1(DIST_NEW) -> Merge/2
  IDVWLK/1 -> If Action Subsystem/1(IDWLK)
  If Action Subsystem1/1(DIST) -> Merge/1
  DIST/1 -> Bus Selector/1, If Action Subsystem/2("DIST ")
  Merge/1 -> DIST_NEW/1
  Bus Selector1/1 -> If Action Subsystem/3(TESUB7)  "<TESUB7_6>"
  [TESUB7] -> Bus Selector1/1

== system Simulink_TEP/Disturbances/Subsystem7/Subsystem2 ==
  IDVWLK : Inport
  DIST : Inport  Port=2
  Bus Selector : BusSelector  OutputSignals=TNEXT
  Bus Selector1 : BusSelector  OutputSignals=TESUB7_7
  Clock : Clock
  If : If  NumInputs=2  IfExpression=u1 == 0  ElseIfExpressions=u1 >= u2  ShowElse=off
  If Action Subsystem : Subsystem  TreatAsAtomicUnit=on
  If Action Subsystem1 : Subsystem  TreatAsAtomicUnit=on
  Merge : Merge
  DIST_NEW : Outport  VectorParamsAs1DForOutWhenUnconnected=off
  wires:
  Clock/1 -> If/1
  If/1 -> If Action Subsystem1/Action
  If/2 -> If Action Subsystem/Action
  Bus Selector/1 -> If/2  "<TNEXT>"
  If Action Subsystem/1(DIST_NEW) -> Merge/2
  IDVWLK/1 -> If Action Subsystem/1(IDWLK)
  If Action Subsystem1/1(DIST) -> Merge/1
  DIST/1 -> Bus Selector/1, If Action Subsystem/2("DIST ")
  Merge/1 -> DIST_NEW/1
  Bus Selector1/1 -> If Action Subsystem/3(TESUB7)  "<TESUB7_7>"
  [TESUB7] -> Bus Selector1/1

== system Simulink_TEP/Disturbances/Subsystem8/Subsystem2 ==
  IDVWLK : Inport
  DIST : Inport  Port=2
  Bus Selector : BusSelector  OutputSignals=TNEXT
  Bus Selector1 : BusSelector  OutputSignals=TESUB7_8
  Clock : Clock
  If : If  NumInputs=2  IfExpression=u1 == 0  ElseIfExpressions=u1 >= u2  ShowElse=off
  If Action Subsystem : Subsystem  TreatAsAtomicUnit=on
  If Action Subsystem1 : Subsystem  TreatAsAtomicUnit=on
  Merge : Merge
  DIST_NEW : Outport  VectorParamsAs1DForOutWhenUnconnected=off
  wires:
  Clock/1 -> If/1
  If/1 -> If Action Subsystem1/Action
  If/2 -> If Action Subsystem/Action
  Bus Selector/1 -> If/2  "<TNEXT>"
  If Action Subsystem/1(DIST_NEW) -> Merge/2
  IDVWLK/1 -> If Action Subsystem/1(IDWLK)
  If Action Subsystem1/1(DIST) -> Merge/1
  DIST/1 -> Bus Selector/1, If Action Subsystem/2("DIST ")
  Merge/1 -> DIST_NEW/1
  Bus Selector1/1 -> If Action Subsystem/3(TESUB7)  "<TESUB7_8>"
  [TESUB7] -> Bus Selector1/1

== system Simulink_TEP/Disturbances/Subsystem9/Subsystem2 ==
  IDVWLK : Inport
  DIST : Inport  Port=2
  Bus Selector : BusSelector  OutputSignals=TNEXT
  Bus Selector1 : BusSelector  OutputSignals=TESUB7_9
  Clock : Clock
  If : If  NumInputs=2  IfExpression=u1 == 0  ElseIfExpressions=u1 >= u2  ShowElse=off
  If Action Subsystem : Subsystem  TreatAsAtomicUnit=on
  If Action Subsystem1 : Subsystem  TreatAsAtomicUnit=on
  Merge : Merge
  DIST_NEW : Outport  VectorParamsAs1DForOutWhenUnconnected=off
  wires:
  Clock/1 -> If/1
  If/1 -> If Action Subsystem1/Action
  If/2 -> If Action Subsystem/Action
  Bus Selector/1 -> If/2  "<TNEXT>"
  If Action Subsystem/1(DIST_NEW) -> Merge/2
  IDVWLK/1 -> If Action Subsystem/1(IDWLK)
  If Action Subsystem1/1(DIST) -> Merge/1
  DIST/1 -> Bus Selector/1, If Action Subsystem/2("DIST ")
  Merge/1 -> DIST_NEW/1
  Bus Selector1/1 -> If Action Subsystem/3(TESUB7)  "<TESUB7_9>"
  [TESUB7] -> Bus Selector1/1

== system Simulink_TEP/Mixing Zone/Holdup of Components in Mixing Zone/Holdup of Vapour Components in the Mixing Zone ==
  YY(28:35) : Inport
  Bus Creator : BusCreator  Inputs=8
  Bus Selector4 : BusSelector  OutputSignals=YY(28),YY(29),YY(30),YY(31),YY(32),YY(33),YY(34),YY(35)
  UCVV(1) Holdup of Component A (Vapour) in Mixing zone lb-mol : Gain
  UCVV(2) Holdup of Component B (Vapour) in Mixing zone lb-mol : Gain
  UCVV(3) Holdup of Component C (Vapour) in Mixing zone lb-mol : Gain
  UCVV(4) Holdup of Component D (Vapour) in Mixing zone lb-mol : Gain
  UCVV(5) Holdup of Component E (Vapour) in Mixing zone lb-mol : Gain
  UCVV(6) Holdup of Component F (Vapour) in Mixing zone lb-mol : Gain
  UCVV(7) Holdup of Component G (Vapour) in Mixing zone lb-mol : Gain
  UCVV(8) Holdup of Component H (Vapour) in Mixing zone lb-mol : Gain
  UCVV : Outport  VectorParamsAs1DForOutWhenUnconnected=off
  wires:
  Bus Selector4/7 -> UCVV(7) Holdup of Component G (Vapour) in Mixing zone lb-mol/1  "<YY(34)>"
  Bus Selector4/2 -> UCVV(2) Holdup of Component B (Vapour) in Mixing zone lb-mol/1  "<YY(29)>"
  Bus Selector4/3 -> UCVV(3) Holdup of Component C (Vapour) in Mixing zone lb-mol/1  "<YY(30)>"
  Bus Selector4/4 -> UCVV(4) Holdup of Component D (Vapour) in Mixing zone lb-mol/1  "<YY(31)>"
  Bus Selector4/5 -> UCVV(5) Holdup of Component E (Vapour) in Mixing zone lb-mol/1  "<YY(32)>"
  Bus Selector4/6 -> UCVV(6) Holdup of Component F (Vapour) in Mixing zone lb-mol/1  "<YY(33)>"
  Bus Selector4/1 -> UCVV(1) Holdup of Component A (Vapour) in Mixing zone lb-mol/1  "<YY(28)>"
  Bus Selector4/8 -> UCVV(8) Holdup of Component H (Vapour) in Mixing zone lb-mol/1  "<YY(35)>"
  YY(28:35)/1 -> Bus Selector4/1
  UCVV(1) Holdup of Component A (Vapour) in Mixing zone lb-mol/1 -> Bus Creator/1  "UCVV(1)"
  UCVV(2) Holdup of Component B (Vapour) in Mixing zone lb-mol/1 -> Bus Creator/2  "UCVV(2)"
  UCVV(3) Holdup of Component C (Vapour) in Mixing zone lb-mol/1 -> Bus Creator/3  "UCVV(3)"
  UCVV(4) Holdup of Component D (Vapour) in Mixing zone lb-mol/1 -> Bus Creator/4  "UCVV(4)"
  UCVV(5) Holdup of Component E (Vapour) in Mixing zone lb-mol/1 -> Bus Creator/5  "UCVV(5)"
  UCVV(6) Holdup of Component F (Vapour) in Mixing zone lb-mol/1 -> Bus Creator/6  "UCVV(6)"
  UCVV(7) Holdup of Component G (Vapour) in Mixing zone lb-mol/1 -> Bus Creator/7  "UCVV(7)"
  UCVV(8) Holdup of Component H (Vapour) in Mixing zone lb-mol/1 -> Bus Creator/8  "UCVV(8)"
  Bus Creator/1 -> UCVV/1

== system Simulink_TEP/Mixing Zone/Holdup of Components in Mixing Zone/Subsystem ==
  Properties of Stream 1 : Inport
  Bus Creator : BusCreator  Inputs=8
  Bus Selector : BusSelector  OutputSignals=FCM(I;1)
  Multiport Selector : dspindex/Multiport Selector  rowsOrCols=Rows  idxCellArray={ 1,2,3,4,5,6,7,8}  idxErrMode=Clip Index
  FCM(I;1) : Outport  VectorParamsAs1DForOutWhenUnconnected=off
  wires:
  Multiport Selector/1 -> Bus Creator/1  "FCM(1;1)"
  Multiport Selector/2 -> Bus Creator/2  "FCM(2;1)"
  Multiport Selector/8 -> Bus Creator/8  "FCM(8;1)"
  Multiport Selector/6 -> Bus Creator/6  "FCM(6;1)"
  Multiport Selector/7 -> Bus Creator/7  "FCM(7;1)"
  Multiport Selector/4 -> Bus Creator/4  "FCM(4;1)"
  Multiport Selector/5 -> Bus Creator/5  "FCM(5;1)"
  Multiport Selector/3 -> Bus Creator/3  "FCM(3;1)"
  Bus Selector/1 -> Multiport Selector/1  "<FCM(I;1)>"
  Properties of Stream 1/1 -> Bus Selector/1
  Bus Creator/1 -> FCM(I;1)/1

== system Simulink_TEP/Mixing Zone/Holdup of Components in Mixing Zone/Subsystem1 ==
  Properties of Stream 2 : Inport
  Bus Creator : BusCreator  Inputs=8
  Bus Selector1 : BusSelector  OutputSignals=FCM(I;2)
  Multiport Selector1 : dspindex/Multiport Selector  rowsOrCols=Rows  idxCellArray={ 1,2,3,4,5,6,7,8}  idxErrMode=Clip Index
  FCM(I;2) : Outport  VectorParamsAs1DForOutWhenUnconnected=off
  wires:
  Multiport Selector1/5 -> Bus Creator/5  "FCM(5;2)"
  Bus Selector1/1 -> Multiport Selector1/1  "<FCM(I;2)>"
  Multiport Selector1/6 -> Bus Creator/6  "FCM(6;2)"
  Multiport Selector1/1 -> Bus Creator/1  "FCM(1;2)"
  Multiport Selector1/2 -> Bus Creator/2  "FCM(2;2)"
  Multiport Selector1/7 -> Bus Creator/7  "FCM(7;2)"
  Multiport Selector1/4 -> Bus Creator/4  "FCM(4;2)"
  Multiport Selector1/8 -> Bus Creator/8  "FCM(8;2)"
  Multiport Selector1/3 -> Bus Creator/3  "FCM(3;2)"
  Properties of Stream 2/1 -> Bus Selector1/1
  Bus Creator/1 -> FCM(I;2)/1

== system Simulink_TEP/Mixing Zone/Holdup of Components in Mixing Zone/Subsystem2 ==
  Bus Creator : BusCreator  Inputs=8
  Bus Selector5 : BusSelector  OutputSignals=signal1.FCM(I;6) = FCM(I;7)
  Multiport Selector4 : dspindex/Multiport Selector  rowsOrCols=Rows  idxCellArray={ 1,2,3,4,5,6,7,8}  idxErrMode=Clip Index
  FCM(I;6) : Outport  VectorParamsAs1DForOutWhenUnconnected=off
  wires:
  Multiport Selector4/6 -> Bus Creator/6  "FCM(6;7)"
  Multiport Selector4/7 -> Bus Creator/7  "FCM(7;7)"
  Multiport Selector4/5 -> Bus Creator/5  "FCM(5;7)"
  Multiport Selector4/4 -> Bus Creator/4  "FCM(4;7)"
  Multiport Selector4/8 -> Bus Creator/8  "FCM(8;7)"
  Multiport Selector4/3 -> Bus Creator/3  "FCM(3;7)"
  Multiport Selector4/2 -> Bus Creator/2  "FCM(2;7)"
  [PropertiesStream6] -> Bus Selector5/1
  Multiport Selector4/1 -> Bus Creator/1  "FCM(1;7)"
  Bus Selector5/1 -> Multiport Selector4/1  "<FCM(I;6) = FCM(I;7)>"
  Bus Creator/1 -> FCM(I;6)/1

== system Simulink_TEP/Mixing Zone/Holdup of Components in Mixing Zone/Subsystem3 ==
  Properties of Stream 3 : Inport
  Bus Creator : BusCreator  Inputs=8
  Bus Selector2 : BusSelector  OutputSignals=FCM(I;3)
  Multiport Selector2 : dspindex/Multiport Selector  rowsOrCols=Rows  idxCellArray={ 1,2,3,4,5,6,7,8}  idxErrMode=Clip Index
  FCM(I;3) : Outport  VectorParamsAs1DForOutWhenUnconnected=off
  wires:
  Multiport Selector2/2 -> Bus Creator/2  "FCM(2;3)"
  Multiport Selector2/4 -> Bus Creator/4  "FCM(4;3)"
  Multiport Selector2/8 -> Bus Creator/8  "FCM(8;3)"
  Bus Selector2/1 -> Multiport Selector2/1  "<FCM(I;3)>"
  Multiport Selector2/7 -> Bus Creator/7  "FCM(7;3)"
  Multiport Selector2/6 -> Bus Creator/6  "FCM(6;3)"
  Multiport Selector2/1 -> Bus Creator/1  "FCM(1;3)"
  Multiport Selector2/3 -> Bus Creator/3  "FCM(3;3)"
  Multiport Selector2/5 -> Bus Creator/5  "FCM(5;3)"
  Properties of Stream 3/1 -> Bus Selector2/1
  Bus Creator/1 -> FCM(I;3)/1

== system Simulink_TEP/Mixing Zone/Holdup of Components in Mixing Zone/Subsystem4 ==
  Properties of Stream 5 : Inport
  Bus Creator : BusCreator  Inputs=8
  Bus Selector3 : BusSelector  OutputSignals=FCM(I;5)
  Multiport Selector3 : dspindex/Multiport Selector  rowsOrCols=Rows  idxCellArray={ 1,2,3,4,5,6,7,8}  idxErrMode=Clip Index
  FCM(I;5) : Outport  VectorParamsAs1DForOutWhenUnconnected=off
  wires:
  Multiport Selector3/6 -> Bus Creator/6  "FCM(6;5)"
  Multiport Selector3/8 -> Bus Creator/8  "FCM(8;5)"
  Multiport Selector3/5 -> Bus Creator/5  "FCM(5;5)"
  Multiport Selector3/2 -> Bus Creator/2  "FCM(2;5)"
  Bus Selector3/1 -> Multiport Selector3/1  "<FCM(I;5)>"
  Multiport Selector3/7 -> Bus Creator/7  "FCM(7;5)"
  Multiport Selector3/4 -> Bus Creator/4  "FCM(4;5)"
  Multiport Selector3/1 -> Bus Creator/1  "FCM(1;5)"
  Multiport Selector3/3 -> Bus Creator/3  "FCM(3;5)"
  Properties of Stream 5/1 -> Bus Selector3/1
  Bus Creator/1 -> FCM(I;5)/1

== system Simulink_TEP/Mixing Zone/Holdup of Components in Mixing Zone/Subsystem5 ==
  Properties of Stream 9 : Inport
  Bus Creator : BusCreator  Inputs=8
  Bus Selector4 : BusSelector  OutputSignals=FCM(I;9)
  Multiport Selector5 : dspindex/Multiport Selector  rowsOrCols=Rows  idxCellArray={ 1,2,3,4,5,6,7,8}  idxErrMode=Clip Index
  FCM(I;9) : Outport  VectorParamsAs1DForOutWhenUnconnected=off
  wires:
  Multiport Selector5/7 -> Bus Creator/7  "FCM(7;9)"
  Multiport Selector5/6 -> Bus Creator/6  "FCM(6;9)"
  Multiport Selector5/8 -> Bus Creator/8  "FCM(8;9)"
  Bus Selector4/1 -> Multiport Selector5/1  "<FCM(I;9)>"
  Multiport Selector5/1 -> Bus Creator/1  "FCM(1;9)"
  Multiport Selector5/2 -> Bus Creator/2  "FCM(2;9)"
  Multiport Selector5/5 -> Bus Creator/5  "FCM(5;9)"
  Multiport Selector5/4 -> Bus Creator/4  "FCM(4;9)"
  Multiport Selector5/3 -> Bus Creator/3  "FCM(3;9)"
  Properties of Stream 9/1 -> Bus Selector4/1
  Bus Creator/1 -> FCM(I;9)/1

== system Simulink_TEP/Mixing Zone/Holdup of Components in Mixing Zone/Vapour Holdup Fraction in the Mxing Zone ==
  UTVV : Inport
  UCVV : Inport  Port=2
  Bus Selector : BusSelector  OutputSignals=UCVV(1),UCVV(2),UCVV(3),UCVV(4),UCVV(5),UCVV(6),UCVV(7),UCVV(8)
  Mux : Mux  Inputs=8
  XVV(1) : Product  Inputs=*/
  XVV(2) : Product  Inputs=*/
  XVV(3) : Product  Inputs=*/
  XVV(4) : Product  Inputs=*/
  XVV(5) : Product  Inputs=*/
  XVV(6) : Product  Inputs=*/
  XVV(7) : Product  Inputs=*/
  XVV(8) : Product  Inputs=*/
  XVV : Outport  VectorParamsAs1DForOutWhenUnconnected=off
  wires:
  XVV(4)/1 -> Mux/4  "XVV(4)"
  UTVV/1 -> XVV(8)/2, XVV(7)/2, XVV(6)/2, XVV(5)/2, XVV(4)/2, XVV(3)/2, XVV(2)/2, XVV(1)/2
  XVV(8)/1 -> Mux/8  "XVV(8)"
  Bus Selector/3 -> XVV(3)/1  "<UCVV(3)>"
  XVV(5)/1 -> Mux/5  "XVV(5)"
  XVV(2)/1 -> Mux/2  "XVV(2)"
  XVV(7)/1 -> Mux/7  "XVV(7)"
  Bus Selector/8 -> XVV(8)/1  "<UCVV(8)>"
  XVV(6)/1 -> Mux/6  "XVV(6)"
  XVV(3)/1 -> Mux/3  "XVV(3)"
  Mux/1 -> XVV/1
  XVV(1)/1 -> Mux/1  "XVV(1)"
  Bus Selector/7 -> XVV(7)/1  "<UCVV(7)>"
  Bus Selector/5 -> XVV(5)/1  "<UCVV(5)>"
  Bus Selector/4 -> XVV(4)/1  "<UCVV(4)>"
  Bus Selector/2 -> XVV(2)/1  "<UCVV(2)>"
  Bus Selector/6 -> XVV(6)/1  "<UCVV(6)>"
  UCVV/1 -> Bus Selector/1
  Bus Selector/1 -> XVV(1)/1  "<UCVV(1)>"

== system Simulink_TEP/Mixing Zone/Holdup of Components in Mixing Zone/YP(28) ==
  FCM(1,1) : Inport
  FCM(1,2) : Inport  Port=2
  FCM(1,3) : Inport  Port=3
  FCM(1,5) : Inport  Port=4
  FCM(1,9) : Inport  Port=5
  FCM(1,6) : Inport  Port=6
  " " : Sum  Inputs=+++++-
  Bus Selector : BusSelector  OutputSignals=FCM(1;1)
  Bus Selector1 : BusSelector  OutputSignals=FCM(1;2)
  Bus Selector2 : BusSelector  OutputSignals=FCM(1;3)
  Bus Selector3 : BusSelector  OutputSignals=FCM(1;5)
  Bus Selector4 : BusSelector  OutputSignals=FCM(1;9)
  Bus Selector5 : BusSelector  OutputSignals=FCM(1;7)
  YP(28) : Integrator  InitialConditionSource=external
  "YY(28) " : Constant  Value=107.7562698
  YY(28) : Outport  VectorParamsAs1DForOutWhenUnconnected=off
  wires:
  "YY(28) "/1 -> YP(28)/2
  FCM(1,3)/1 -> Bus Selector2/1
  FCM(1,2)/1 -> Bus Selector1/1
  " "/1 -> YP(28)/1
  YP(28)/1 -> YY(28)/1
  FCM(1,5)/1 -> Bus Selector3/1
  FCM(1,9)/1 -> Bus Selector4/1
  FCM(1,6)/1 -> Bus Selector5/1
  FCM(1,1)/1 -> Bus Selector/1
  Bus Selector/1 -> " "/1  "<FCM(1;1)>"
  Bus Selector1/1 -> " "/2  "<FCM(1;2)>"
  Bus Selector2/1 -> " "/3  "<FCM(1;3)>"
  Bus Selector3/1 -> " "/4  "<FCM(1;5)>"
  Bus Selector4/1 -> " "/5  "<FCM(1;9)>"
  Bus Selector5/1 -> " "/6  "<FCM(1;7)>"
